simulink model "Lab3_Topolnitskii_velocity"  (R2021a)
settings: Solver=VariableStepAuto  StartTime=0.0  StopTime=1  RelTol=1e-3
undefined symbols (not defined in the file): irb140, J, Ki, Kv, motor_const, tau_m
libraries: roblocks x6, simulink x1
settings Model: Creator=SPb19  LastModifiedBy=Insight

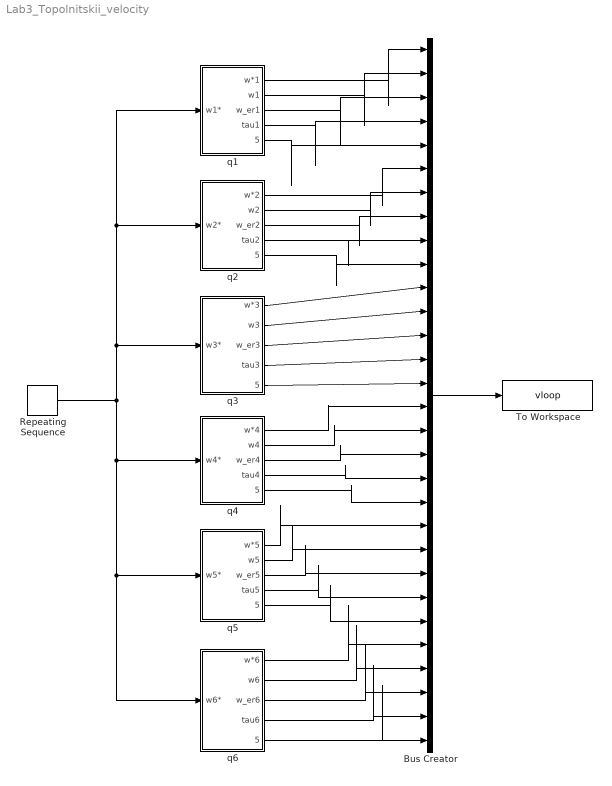
== system Lab3_Topolnitskii_velocity ==
  Bus Creator : BusCreator  Inputs=30
  Repeating Sequence : simulink/Sources/Repeating Sequence  rep_seq_t=[0 1 3 5 7]/10  rep_seq_y=[0 50 45 0 0]
  To Workspace : ToWorkspace  VariableName=vloop  SaveFormat=Structure With Time  SampleTime=-1
  q1 : Subsystem
  q2 : Subsystem
  q3 : Subsystem
  q4 : Subsystem
  q5 : Subsystem
  q6 : Subsystem
  wires:
  Repeating Sequence/1 -> q1/1(w1*), q2/1(w2*), q3/1(w3*), q6/1(w6*), q5/1(w5*), q4/1(w4*)
  Bus Creator/1 -> To Workspace/1
  q1/1(w*1) -> Bus Creator/1
  q1/2(w1) -> Bus Creator/2
  q1/3(w_er1) -> Bus Creator/3
  q1/4(tau1) -> Bus Creator/4
  q1/5(integral1) -> Bus Creator/5
  q2/1(w*2) -> Bus Creator/6
  q2/2(w2) -> Bus Creator/7
  q2/3(w_er2) -> Bus Creator/8
  q2/4(tau2) -> Bus Creator/9
  q2/5(integral2) -> Bus Creator/10
  q3/1(w*3) -> Bus Creator/11
  q3/2(w3) -> Bus Creator/12
  q3/3(w_er3) -> Bus Creator/13
  q3/4(tau3) -> Bus Creator/14
  q3/5(integral3) -> Bus Creator/15
  q4/1(w*4) -> Bus Creator/16
  q4/2(w4) -> Bus Creator/17
  q4/3(w_er4) -> Bus Creator/18
  q4/4(tau4) -> Bus Creator/19
  q4/5(integral4) -> Bus Creator/20
  q5/1(w*5) -> Bus Creator/21
  q5/2(w5) -> Bus Creator/22
  q5/3(w_er5) -> Bus Creator/23
  q5/4(tau5) -> Bus Creator/24
  q5/5(integral5) -> Bus Creator/25
  q6/1(w*6) -> Bus Creator/26
  q6/2(w6) -> Bus Creator/27
  q6/3(w_er6) -> Bus Creator/28
  q6/4(tau6) -> Bus Creator/29
  q6/5(integral6) -> Bus Creator/30

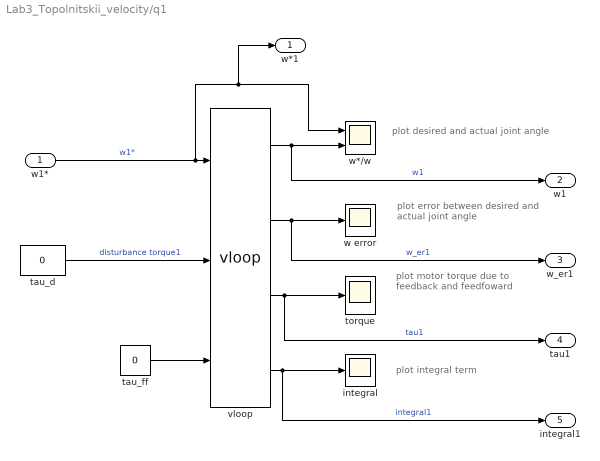
== system Lab3_Topolnitskii_velocity/q1 ==
  note: plot integral term
  note: plot motor torque due
      | to feedback and feedfoward
  note: plot desired and actual joint angle
  note: plot error between desired and
      | actual joint angle
  w1* : Inport
  "integral " : Scope
  tau_d : Constant  Value=0
  tau_ff : Constant  Value=0
  torque : Scope
  vloop : roblocks/Arm/vloop  J=J(1)  B=irb140.links(1, 1).B  Km=motor_const(1)  tau_max=tau_m(1)  Kv=Kv(1)  Ki=Ki(1)  T=0.0001
  w error : Scope
  w*/w : Scope  NumInputPorts=2
  w*1 : Outport
  w1 : Outport  Port=2
  w_er1 : Outport  Port=3
  tau1 : Outport  Port=4
  integral1 : Outport  Port=5
  wires:
  tau_d/1 -> vloop/2  "disturbance torque1"
  w1*/1 -> w*1/1, w*/w/1, vloop/1  "w1*"
  tau_ff/1 -> vloop/3
  vloop/2 -> w_er1/1, w error/1  "w_er1"
  vloop/4 -> integral1/1, "integral "/1  "integral1"
  vloop/1 -> w1/1, w*/w/2  "w1"
  vloop/3 -> tau1/1, torque/1  "tau1"

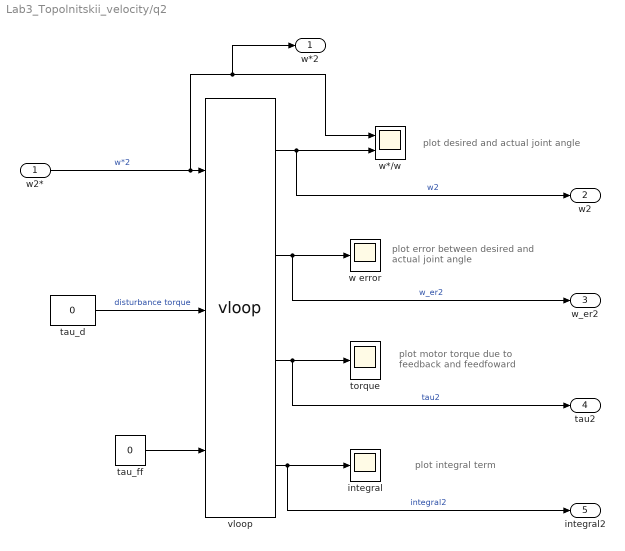
== system Lab3_Topolnitskii_velocity/q2 ==
  note: plot integral term
  note: plot motor torque due
      | to feedback and feedfoward
  note: plot desired and actual joint angle
  note: plot error between desired and
      | actual joint angle
  w2* : Inport
  "integral " : Scope
  tau_d : Constant  Value=0
  tau_ff : Constant  Value=0
  torque : Scope
  vloop : roblocks/Arm/vloop  J=J(2)  B=irb140.links(1, 2).B  Km=motor_const(2)  tau_max=tau_m(2)  Kv=Kv(2)  Ki=Ki(2)  T=0.001
  w error : Scope
  w*/w : Scope  NumInputPorts=2
  w*2 : Outport
  w2 : Outport  Port=2
  w_er2 : Outport  Port=3
  tau2 : Outport  Port=4
  integral2 : Outport  Port=5
  wires:
  tau_d/1 -> vloop/2  "disturbance torque"
  w2*/1 -> w*2/1, w*/w/1, vloop/1  "w*2"
  tau_ff/1 -> vloop/3
  vloop/2 -> w_er2/1, w error/1  "w_er2"
  vloop/4 -> integral2/1, "integral "/1  "integral2"
  vloop/1 -> w2/1, w*/w/2  "w2"
  vloop/3 -> tau2/1, torque/1  "tau2"

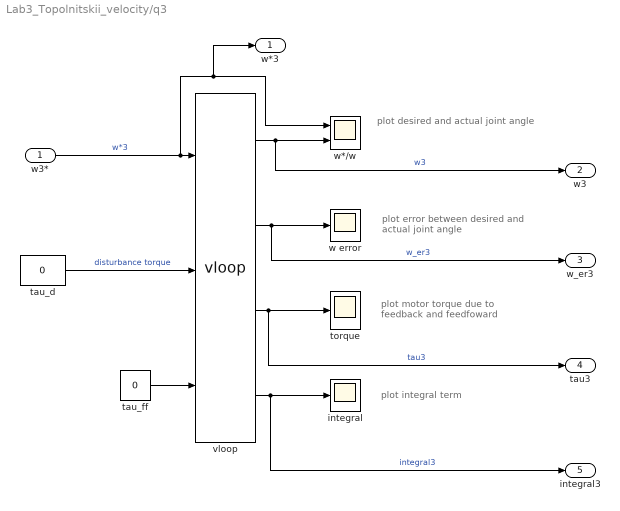
== system Lab3_Topolnitskii_velocity/q3 ==
  note: plot integral term
  note: plot motor torque due
      | to feedback and feedfoward
  note: plot desired and actual joint angle
  note: plot error between desired and
      | actual joint angle
  w3* : Inport
  "integral " : Scope
  tau_d : Constant  Value=0
  tau_ff : Constant  Value=0
  torque : Scope
  vloop : roblocks/Arm/vloop  J=J(3)  B=irb140.links(1, 3).B  Km=motor_const(3)  tau_max=tau_m(3)  Kv=Kv(3)  Ki=Ki(3)  T=0.001
  w error : Scope
  w*/w : Scope  NumInputPorts=2
  w*3 : Outport
  w3 : Outport  Port=2
  w_er3 : Outport  Port=3
  tau3 : Outport  Port=4
  integral3 : Outport  Port=5
  wires:
  tau_d/1 -> vloop/2  "disturbance torque"
  w3*/1 -> w*3/1, w*/w/1, vloop/1  "w*3"
  tau_ff/1 -> vloop/3
  vloop/2 -> w_er3/1, w error/1  "w_er3"
  vloop/4 -> integral3/1, "integral "/1  "integral3"
  vloop/1 -> w3/1, w*/w/2  "w3"
  vloop/3 -> tau3/1, torque/1  "tau3"

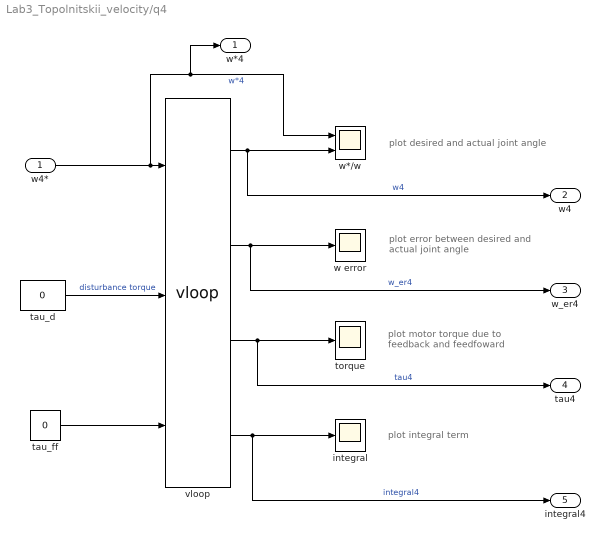
== system Lab3_Topolnitskii_velocity/q4 ==
  note: plot integral term
  note: plot motor torque due
      | to feedback and feedfoward
  note: plot desired and actual joint angle
  note: plot error between desired and
      | actual joint angle
  w4* : Inport
  "integral " : Scope
  tau_d : Constant  Value=0
  tau_ff : Constant  Value=0
  torque : Scope
  vloop : roblocks/Arm/vloop  J=J(4)  B=irb140.links(1, 4).B  Km=motor_const(4)  tau_max=tau_m(4)  Kv=Kv(4)  Ki=Ki(4)  T=0.001
  w error : Scope
  w*/w : Scope  NumInputPorts=2
  w*4 : Outport
  w4 : Outport  Port=2
  w_er4 : Outport  Port=3
  tau4 : Outport  Port=4
  integral4 : Outport  Port=5
  wires:
  tau_d/1 -> vloop/2  "disturbance torque"
  w4*/1 -> w*4/1, w*/w/1, vloop/1  "w*4"
  tau_ff/1 -> vloop/3
  vloop/2 -> w_er4/1, w error/1  "w_er4"
  vloop/4 -> integral4/1, "integral "/1  "integral4"
  vloop/1 -> w4/1, w*/w/2  "w4"
  vloop/3 -> tau4/1, torque/1  "tau4"

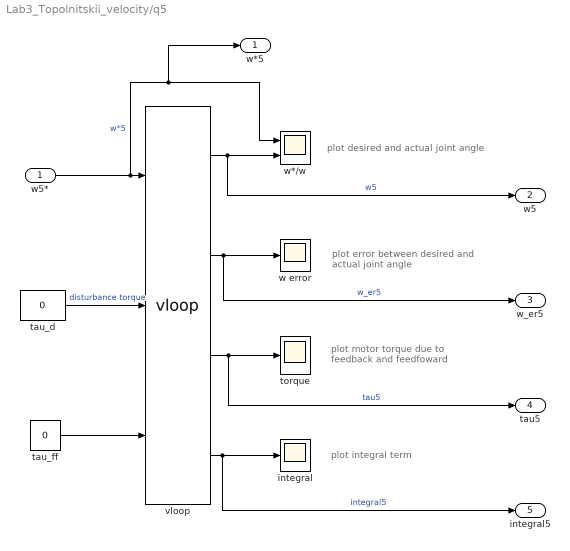
== system Lab3_Topolnitskii_velocity/q5 ==
  note: plot integral term
  note: plot motor torque due
      | to feedback and feedfoward
  note: plot desired and actual joint angle
  note: plot error between desired and
      | actual joint angle
  w5* : Inport
  "integral " : Scope
  tau_d : Constant  Value=0
  tau_ff : Constant  Value=0
  torque : Scope
  vloop : roblocks/Arm/vloop  J=J(5)  B=irb140.links(1, 5).B  Km=motor_const(5)  tau_max=tau_m(5)  Kv=Kv(5)  Ki=Ki(5)  T=0.001
  w error : Scope
  w*/w : Scope  NumInputPorts=2
  w*5 : Outport
  w5 : Outport  Port=2
  w_er5 : Outport  Port=3
  tau5 : Outport  Port=4
  integral5 : Outport  Port=5
  wires:
  tau_d/1 -> vloop/2  "disturbance torque"
  w5*/1 -> w*5/1, w*/w/1, vloop/1  "w*5"
  tau_ff/1 -> vloop/3
  vloop/2 -> w_er5/1, w error/1  "w_er5"
  vloop/4 -> integral5/1, "integral "/1  "integral5"
  vloop/1 -> w5/1, w*/w/2  "w5"
  vloop/3 -> tau5/1, torque/1  "tau5"

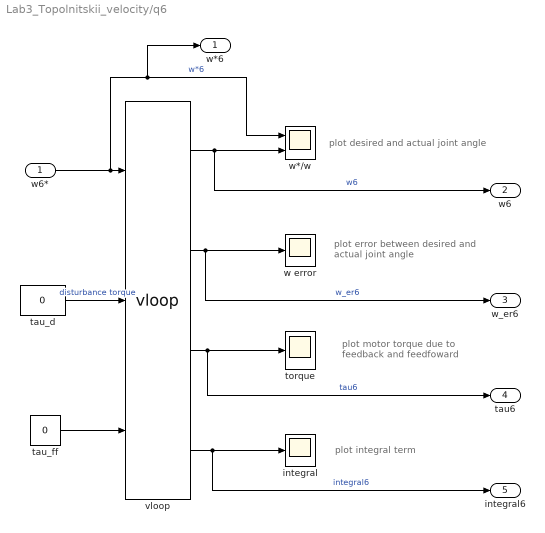
== system Lab3_Topolnitskii_velocity/q6 ==
  note: plot integral term
  note: plot motor torque due
      | to feedback and feedfoward
  note: plot desired and actual joint angle
  note: plot error between desired and
      | actual joint angle
  w6* : Inport
  "integral " : Scope
  tau_d : Constant  Value=0
  tau_ff : Constant  Value=0
  torque : Scope
  vloop : roblocks/Arm/vloop  J=J(6)  B=irb140.links(1, 6).B  Km=motor_const(6)  tau_max=tau_m(6)  Kv=Kv(6)  Ki=Ki(6)  T=0.001
  w error : Scope
  w*/w : Scope  NumInputPorts=2
  w*6 : Outport
  w6 : Outport  Port=2
  w_er6 : Outport  Port=3
  tau6 : Outport  Port=4
  integral6 : Outport  Port=5
  wires:
  tau_d/1 -> vloop/2  "disturbance torque"
  w6*/1 -> w*6/1, w*/w/1, vloop/1  "w*6"
  tau_ff/1 -> vloop/3
  vloop/2 -> w_er6/1, w error/1  "w_er6"
  vloop/4 -> integral6/1, "integral "/1  "integral6"
  vloop/1 -> w6/1, w*/w/2  "w6"
  vloop/3 -> tau6/1, torque/1  "tau6"
